simulink model "StepbyStepMotorControl_Slave_SM"  (R2018b)
settings: Solver=FixedStepDiscrete  StartTime=0.0  StopTime=10.0  FixedStep=0.1  RelTol=1e-3
InitFcn:
  | mbd_s32k14_consistency_checks(bdroot(gcs));
undefined symbols (not defined in the file): A10, AD12, AD6, AD7, Aligned, B1, B10, B8, C10, C7, C8, C9, Center, D1, D2, D8, External, G2, G3, G6, H8, K10, PTA2, PTA3, PTB10, PTB11, PTB12, PTB8, PTB9, PTC10, PTC11, PTC14, PTC6, PTC7, PTD1, PTD15, PTD16, PTD4, PTE4, PTE5, TRGMUX_PDB_TRIG
libraries: mbd_s32k14_ec_toolbox x26, simulink x2
settings Model: Creator=srjos  LastModifiedBy=srjos
settings DataIOCC: ExternalInput=off  InitialState=off  SaveOutput=off  SignalLogging=off  SaveTime=off
settings OptimizationCC: DefaultParameterBehavior=Inlined  EnhancedBackFolding=on  PassReuseOutputArgsAs=Individual arguments  OptimizeBlockOrder=speed  DifferentSizesBufferReuse=on  OptimizationCustomize=off
settings DebuggingCC: InheritedTsInSrcMsg=none  SingleTaskRateTransMsg=error  ParameterTunabilityLossMsg=error  UnconnectedInputMsg=error  UnconnectedOutputMsg=error  UnconnectedLineMsg=error  UnknownTsInhSupMsg=error
settings HardwareCC: ProdBitPerPointer=32  ProdBitPerSizeT=32  ProdBitPerPtrDiffT=32  ProdLargestAtomicInteger=Long  ProdLargestAtomicFloat=Double  ProdWordSize=32  ProdHWDeviceType=ARM Compatible->ARM Cortex
settings SFSimCC: MATLABDynamicMemAlloc=off
settings RTWCC: SystemTargetFile=mbd_s32k14.tlc  MakeCommand=mbd_s32k14_make_rtw COPY_MDLREF_INCLUDES=0  TemplateMakefile=mbd_s32k14.tmf  Description=Model Based Design Toolbox S32K14x Code Generation Target  GenerateReport=on  IncludeHyperlinkInReport=on  LaunchReport=on  GenerateTraceInfo=on  GenerateTraceReport=on  GenerateTraceReportSl=on  GenerateTraceReportSf=on  GenerateTraceReportEml=on
settings CodeAppCC: ForceParamTrailComments=on  IgnoreCustomStorageClasses=off  OperatorAnnotations=on  SimulinkDataObjDesc=on  SFDataObjDesc=on  InsertBlockDesc=on
settings STFCustomTargetCC: TargetLangStandard=C99 (ISO)  MultiwordLength=256  CombineOutputUpdateFcns=on  ERTCustomFileBanners=on  SupportContinuousTime=off  SupportNonInlinedSFcns=off  RemoveResetFunc=on  MATLABClassNameForMDSCustomization=Simulink.SoftwareTarget.ERTCustomization  SystemTargetFile=mbd_s32k14.tlc
settings ERTTargetCC: TargetLangStandard=C99 (ISO)  ParMdlRefBuildCompliant=off  CompOptLevelCompliant=off  ConcurrentExecutionCompliant=off  ModelStepFunctionPrototypeControlCompliant=off  CPPClassGenCompliant=off  UseToolchainInfoCompliant=off  InlinedParameterPlacement=NonHierarchical  ERTCustomFileTemplate=example_file_process.tlc

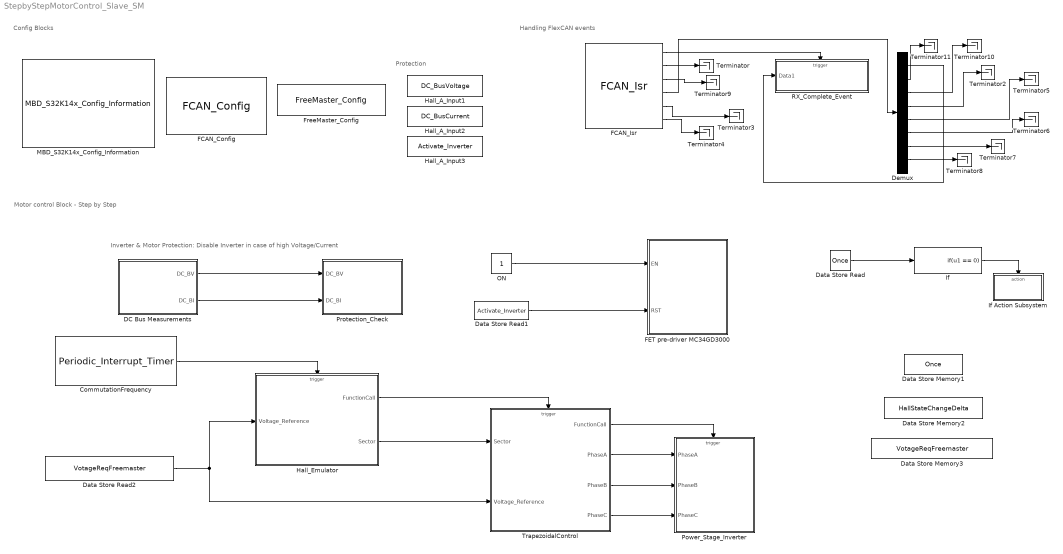
== system StepbyStepMotorControl_Slave_SM ==
  note: Config Blocks
  note: Motor control Block - Step by Step
  note: Inverter & Motor Protection: Disable Inverter in case of high Voltage/Current
  note: Protection
  note: Handling FlexCAN events
  CommutationFrequency : mbd_s32k14_ec_toolbox/S32K14x/Utility Blocks/Periodic_Interrupt_Timer  Priority=1  channel=1  chainCh=off  period=20000  prio=10  startCounter=on
  DC Bus Measurements : Subsystem  Priority=6
  Data Store Memory1 : DataStoreMemory  DataStoreName=Once  ReadBeforeWriteMsg=warning  WriteAfterWriteMsg=warning  WriteAfterReadMsg=warning  ShowAdditionalParam=off  OutDataTypeStr=uint32
  Data Store Memory2 : DataStoreMemory  DataStoreName=HallStateChangeDelta  ReadBeforeWriteMsg=warning  WriteAfterWriteMsg=warning  WriteAfterReadMsg=warning  ShowAdditionalParam=off  OutDataTypeStr=uint16
      settings: RTWStateStorageClass=ExportedGlobal
  Data Store Memory3 : DataStoreMemory  DataStoreName=VotageReqFreemaster  ReadBeforeWriteMsg=warning  WriteAfterWriteMsg=warning  WriteAfterReadMsg=warning  ShowAdditionalParam=off  OutDataTypeStr=int16
      settings: RTWStateStorageClass=ExportedGlobal
  Data Store Read : DataStoreRead  DataStoreName=Once
  Data Store Read1 : DataStoreRead  DataStoreName=Activate_Inverter
  Data Store Read2 : DataStoreRead  DataStoreName=VotageReqFreemaster
  Demux : Demux  Outputs=8
  FCAN_Config : mbd_s32k14_ec_toolbox/S32K14x/Communication Blocks/Flex CAN Blocks/FCAN_Config  Priority=1  can_instance=0  can_mode=Normal mode  can_max_num_mb=16  can_rx=PTE4 : [9] : [6] : [D1]  can_tx=PTE5 : [8] : [5] : [D2]  show_adv_opts=on  can_clk_src=Peripheral clock  can_presdiv=9  can_rjw=0  can_pseg1=3  can_pseg2=3  can_propseg=6  can_cbt_presdiv=9  can_cbt_rjw=0  can_cbt_pseg1=3  can_cbt_pseg2=3  can_cbt_propseg=6  can_fd_enable=on  can_payload=8  can_rxfifo_enable=off  can_fifo_id_filter_extended=off  can_fifo_id_filter_remote=off  can_num_id_filters=8  can_fifo_id_format=A  can_fifo_id_filter={'0x0', '0x0', '0x0', '0x0', '0x0', '0x0', '0x0', '0x0'}  can_pn_enable=off  can_wakeup_match=off  can_wakeup_timeout=off  can_timeout_en=off  can_match_timeout=1  can_multiple_matches_en=off  can_num_matches=1  can_idfilter_extendedid=off  can_idfilter_remoteframe=off  can_idfilter_type=Match exact  can_idfilter_id1=0  can_idfilter_id2=0  can_payloadfilter_enable=off  can_payloadfilter_dlclow=0  can_payloadfilter_dlchigh=0  can_payloadfilter_type=Match exact  can_payloadfilter_payload1_b0=0  can_payloadfilter_payload1_b1=0  can_payloadfilter_payload1_b2=0  can_payloadfilter_payload1_b3=0  can_payloadfilter_payload1_b4=0  can_payloadfilter_payload1_b5=0  can_payloadfilter_payload1_b6=0  can_payloadfilter_payload1_b7=0  can_payloadfilter_payload2_b0=0  can_payloadfilter_payload2_b1=0  can_payloadfilter_payload2_b2=0  can_payloadfilter_payload2_b3=0  can_payloadfilter_payload2_b4=0  can_payloadfilter_payload2_b5=0  can_payloadfilter_payload2_b6=0  can_payloadfilter_payload2_b7=0
  FCAN_Isr : mbd_s32k14_ec_toolbox/S32K14x/Communication Blocks/Flex CAN Blocks/FCAN_Isr  can_instance=0  can_event=Rx Complete
  FET pre-driver MC34GD3000 : Subsystem
  FreeMaster_Config : mbd_s32k14_ec_toolbox/S32K14x/Utility Blocks/FreeMaster_Config  interface=UART1  baudrate=115200  rxd=PTC6 : [81] : [52] : [C7]  txd=PTC7 : [80] : [51] : [B8]  mode=Short Interrupt  isr_prio=15  show_adv_opts=off  use_scope=on  max_scope_vars=8  use_recorder=on  max_rec_vars=8  rec_buff_size=1024  rec_timebase=0 milliseconds  comm_buffer_size_auto=on  comm_buffer_size=255  comm_rqueue_size_default=on  comm_rqueue_size=32
  Hall_A_Input1 : DataStoreMemory  DataStoreName=DC_BusVoltage  ReadBeforeWriteMsg=warning  WriteAfterWriteMsg=warning  WriteAfterReadMsg=warning  ShowAdditionalParam=off  OutDataTypeStr=single
  Hall_A_Input2 : DataStoreMemory  DataStoreName=DC_BusCurrent  ReadBeforeWriteMsg=warning  WriteAfterWriteMsg=warning  WriteAfterReadMsg=warning  ShowAdditionalParam=off  OutDataTypeStr=single
  Hall_A_Input3 : DataStoreMemory  DataStoreName=Activate_Inverter  ReadBeforeWriteMsg=warning  WriteAfterWriteMsg=warning  WriteAfterReadMsg=warning  ShowAdditionalParam=off  OutDataTypeStr=boolean
  Hall_Emulator : Subsystem
      settings: PropExecContextOutsideSubsystem=on  RTWSystemCode=Nonreusable function
  If : If  IfExpression=u1 == 0  ShowElse=off
  If Action Subsystem : Subsystem  TreatAsAtomicUnit=on
  MBD_S32K14x_Config_Information : mbd_s32k14_ec_toolbox/S32K14x/MBD_S32K14x_Config_Information  disp_str=|  config_params=[]
      | Target : S32K144-64KB_SRAM
      | Package : 100-pin
      | System clock : 80 MHz
      | XTAL clock : External 8 MHz
      | Compiler : GCC
      | Target Type : FLASH
      | Download Code after build : (OpenSDA: E)
      | Step Tick Interrupt Priority : 15
  ON : Constant  OutDataTypeStr=boolean
  Power_Stage_Inverter : Subsystem  TreatAsAtomicUnit=on
      settings: RTWSystemCode=Nonreusable function
  Protection_Check : Subsystem
  RX_Complete_Event : Subsystem  TreatAsAtomicUnit=on
      settings: RTWSystemCode=Nonreusable function
  Terminator{,2..11} (11 alike) : Terminator
  TrapezoidalControl : Subsystem
      settings: RTWSystemCode=Nonreusable function
  wires:
  DC Bus Measurements/2(DC_BI) -> Protection_Check/2(DC_BI)
  CommutationFrequency/1 -> Hall_Emulator/Trigger
  Data Store Read1/1 -> FET pre-driver MC34GD3000/2(RST)
  DC Bus Measurements/1(DC_BV) -> Protection_Check/1(DC_BV)
  TrapezoidalControl/1(FunctionCall) -> Power_Stage_Inverter/Trigger
  TrapezoidalControl/2(PhaseA) -> Power_Stage_Inverter/1(PhaseA)
  Data Store Read2/1 -> TrapezoidalControl/2(Voltage_Reference), Hall_Emulator/1(Voltage_Reference)
  ON/1 -> FET pre-driver MC34GD3000/1(EN)
  TrapezoidalControl/4(PhaseC) -> Power_Stage_Inverter/3(PhaseC)
  Hall_Emulator/1(FunctionCall) -> TrapezoidalControl/Trigger
  TrapezoidalControl/3(PhaseB) -> Power_Stage_Inverter/2(PhaseB)
  Hall_Emulator/2(Sector) -> TrapezoidalControl/1(Sector)
  Demux/4 -> Terminator2/1
  FCAN_Isr/4 -> Demux/1
  FCAN_Isr/2 -> Terminator/1
  FCAN_Isr/6 -> Terminator4/1
  FCAN_Isr/1 -> RX_Complete_Event/Trigger
  Demux/5 -> Terminator5/1
  Demux/7 -> Terminator7/1
  Demux/1 -> RX_Complete_Event/1(Data1)
  FCAN_Isr/3 -> Terminator9/1
  Demux/6 -> Terminator6/1
  Demux/2 -> Terminator11/1
  Demux/3 -> Terminator10/1
  Demux/8 -> Terminator8/1
  FCAN_Isr/5 -> Terminator3/1
  If/1 -> If Action Subsystem/Action
  Data Store Read/1 -> If/1

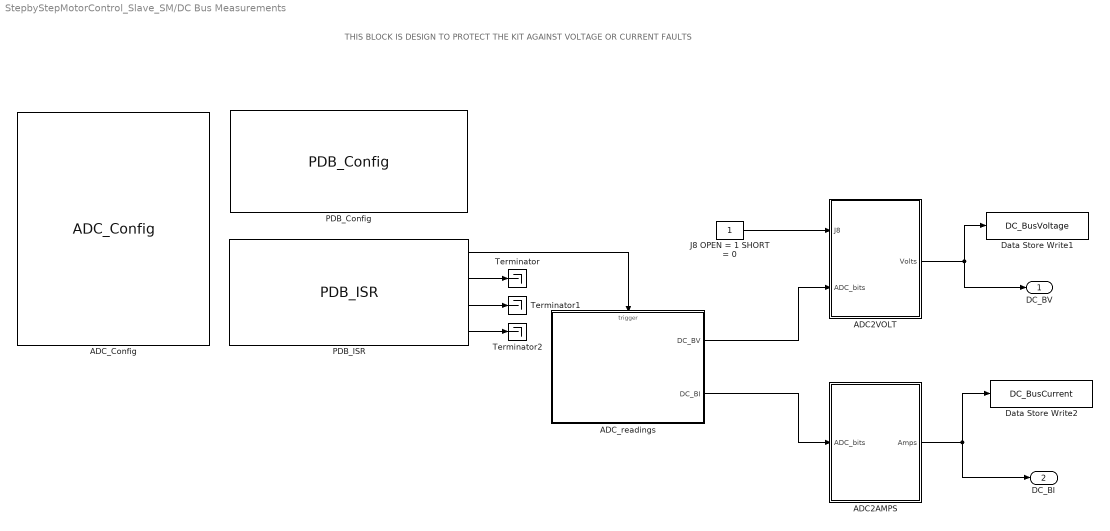
== system StepbyStepMotorControl_Slave_SM/DC Bus Measurements ==
  note: THIS BLOCK IS DESIGN TO PROTECT THE KIT AGAINST VOLTAGE OR CURRENT FAULTS
  ADC2AMPS : Subsystem
  ADC2VOLT : Subsystem
  ADC_Config : mbd_s32k14_ec_toolbox/S32K14x/Motor Control Blocks/ADC Blocks/ADC_Config  Priority=1  instance=1  mode=12-bit conversion  smplts=64  adiclk=alternate clock 1  adiv=input clock  show_adv_opts=on  pretrgsel=PDB pre-trigger  swpretrg=Disabled  adtrg=hardware  trgsel=PDB output  refsel=Vrefh and Vrefl  acfe=off  acfgt=off  acren=off  cv1=0  cv2=0  adco=off  avge=off  avgs=16 samples
  ADC_readings : Subsystem  TreatAsAtomicUnit=on
      settings: RTWSystemCode=Nonreusable function
  Data Store Write1 : DataStoreWrite  DataStoreName=DC_BusVoltage
  Data Store Write2 : DataStoreWrite  DataStoreName=DC_BusCurrent
  J8 OPEN = 1 SHORT = 0 : Constant  OutDataTypeStr=boolean
  PDB_Config : mbd_s32k14_ec_toolbox/S32K14x/Motor Control Blocks/PDB Blocks/PDB_Config  Priority=1  pdbModule=1  regScCont=Continuous  regScTrgsel=External (TRGMUX_PDB_TRIG)  trgMuxSel=FTM3 External Trigger  regModModulus=10000  regScPrescaler=8  regScMult=1  regPoenPoen0=off  regPo0DlyDly1=0  regPo0DlyDly2=1000  show_adv_opts=off  regCh0C1En0=on  regCh0C1En1=on  regCh0C1En2=off  regCh0C1En3=off  regCh0C1En4=off  regCh0C1En5=off  regCh0C1En6=off  regCh0C1En7=off  regCh0C1Bb0=off  regCh0C1Bb1=off  regCh0C1Bb2=off  regCh0C1Bb3=off  regCh0C1Bb4=off  regCh0C1Bb5=off  regCh0C1Bb6=off  regCh0C1Bb7=off  regCh0C1Tos0=Pre-trigger is in delay mode  regCh0C1Tos1=Pre-trigger is in delay mode  regCh0C1Tos2=Pre-trigger is in delay mode  regCh0C1Tos3=Pre-trigger is in delay mode  regCh0C1Tos4=Pre-trigger is in delay mode  regCh0C1Tos5=Pre-trigger is in delay mode  regCh0C1Tos6=Pre-trigger is in delay mode  regCh0C1Tos7=Pre-trigger is in delay mode  regCh0DlyDly0=300  regCh0DlyDly1=400  regCh0DlyDly2=100  regCh0DlyDly3=480  regCh0DlyDly4=600  regCh0DlyDly5=720  regCh0DlyDly6=840  regCh0DlyDly7=960  regCh1C1En0=off  regCh1C1En1=off  regCh1C1En2=off  regCh1C1En3=off  regCh1C1En4=off  regCh1C1En5=off  regCh1C1En6=off  regCh1C1En7=off  regCh1C1Bb0=off  regCh1C1Bb1=off  regCh1C1Bb2=off  regCh1C1Bb3=off  regCh1C1Bb4=off  regCh1C1Bb5=off  regCh1C1Bb6=off  regCh1C1Bb7=off  regCh1C1Tos0=Pre-trigger is in delay mode  regCh1C1Tos1=Pre-trigger is in delay mode  regCh1C1Tos2=Pre-trigger is in delay mode  regCh1C1Tos3=Pre-trigger is in delay mode  regCh1C1Tos4=Pre-trigger is in delay mode  regCh1C1Tos5=Pre-trigger is in delay mode  regCh1C1Tos6=Pre-trigger is in delay mode  regCh1C1Tos7=Pre-trigger is in delay mode  regCh1DlyDly0=100  regCh1DlyDly1=200  regCh1DlyDly2=300  regCh1DlyDly3=400  regCh1DlyDly4=500  regCh1DlyDly5=600  regCh1DlyDly6=700  regCh1DlyDly7=800
  PDB_ISR : mbd_s32k14_ec_toolbox/S32K14x/Motor Control Blocks/PDB Blocks/PDB_ISR  Priority=2  pdbModule=1  prioInterrupt=5  regScPdbie=on  regScPdbeie=off  regIdlyIdly=0
  Terminator : Terminator
  Terminator1 : Terminator
  Terminator2 : Terminator
  DC_BV : Outport
  DC_BI : Outport  Port=2
  wires:
  PDB_ISR/2 -> Terminator/1
  PDB_ISR/4 -> Terminator2/1
  PDB_ISR/3 -> Terminator1/1
  PDB_ISR/1 -> ADC_readings/Trigger
  ADC2VOLT/1(Volts) -> DC_BV/1, Data Store Write1/1
  J8 OPEN = 1 SHORT = 0/1 -> ADC2VOLT/1(J8)
  ADC_readings/1(DC_BV) -> ADC2VOLT/2(ADC_bits)
  ADC2AMPS/1(Amps) -> Data Store Write2/1, DC_BI/1
  ADC_readings/2(DC_BI) -> ADC2AMPS/1(ADC_bits)

== system StepbyStepMotorControl_Slave_SM/FET pre-driver MC34GD3000 ==
  EN : Inport
  RST : Inport  Port=2
  GD3000_EN : mbd_s32k14_ec_toolbox/S32K14x/Peripheral Interface Blocks/Digital_Output  gpio_pin=PTA2 : [73] : [48] : [C10]  port=A  pin=2  drive_strength=High  slew_rate=Fast
  GD3000_RST : mbd_s32k14_ec_toolbox/S32K14x/Peripheral Interface Blocks/Digital_Output  gpio_pin="PTA3 : [72] : [47]  : [D8]"  port=A  pin=3  drive_strength=High  slew_rate=Fast
  wires:
  EN/1 -> GD3000_EN/1
  RST/1 -> GD3000_RST/1

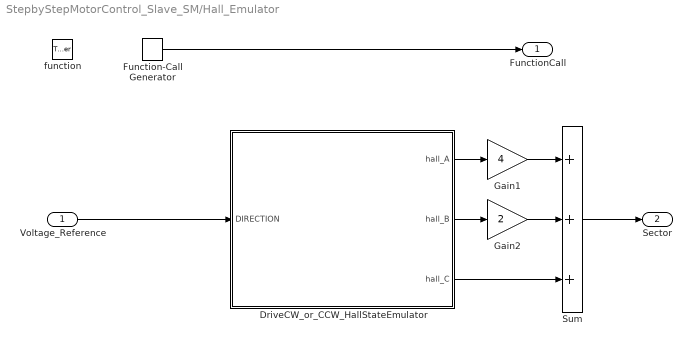
== system StepbyStepMotorControl_Slave_SM/Hall_Emulator ==
  Voltage_Reference : Inport
  function : TriggerPort  TriggerType=function-call  VariantControl=(inherit)
  DriveCW_or_CCW_HallStateEmulator : Stateflow chart  TreatAsAtomicUnit=on
  Function-Call Generator : simulink/Ports & Subsystems/Function-Call Generator  sample_time=-1  numberOfIterations=1
  Gain1 : Gain  Gain=4  OutDataTypeStr=uint8  ParamDataTypeStr=Inherit: Same as input
  Gain2 : Gain  Gain=2  OutDataTypeStr=uint8  ParamDataTypeStr=Inherit: Same as input
  Sum : Sum  Inputs=+++  AccumDataTypeStr=uint8  OutDataTypeStr=uint8
  FunctionCall : Outport
  Sector : Outport  Port=2  OutDataTypeStr=uint8
  wires:
  Function-Call Generator/1 -> FunctionCall/1
  Gain1/1 -> Sum/1
  DriveCW_or_CCW_HallStateEmulator/1(hall_A) -> Gain1/1
  Gain2/1 -> Sum/2
  DriveCW_or_CCW_HallStateEmulator/3(hall_C) -> Sum/3
  DriveCW_or_CCW_HallStateEmulator/2(hall_B) -> Gain2/1
  Sum/1 -> Sector/1
  Voltage_Reference/1 -> DriveCW_or_CCW_HallStateEmulator/1(DIRECTION)

== system StepbyStepMotorControl_Slave_SM/If Action Subsystem ==
  Action Port : ActionPort  ActionType=then
  Constant : Constant  OutDataTypeStr=uint32
  Data Store Write : DataStoreWrite  DataStoreName=Once
  FCAN_Receive_ID_0x3FF : mbd_s32k14_ec_toolbox/S32K14x/Communication Blocks/Flex CAN Blocks/FCAN_Receive  can_instance=0  can_mode=Non-blocking  can_timeout_ms=0  can_mb_idx=14  can_extended_id=off  can_is_remote=off  can_id=3FF  can_msg_mask=FFFFFFFF  show_adv_opts=on  can_use_rxfifo=off  can_fd_enable=on
  wires:
  Constant/1 -> Data Store Write/1

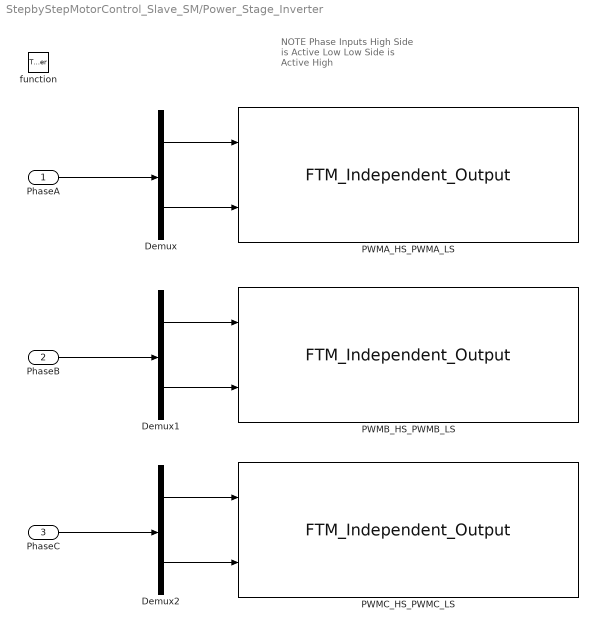
== system StepbyStepMotorControl_Slave_SM/Power_Stage_Inverter ==
  note: NOTE
      | Phase Inputs
      | High Side is Active Low
      | Low Side is Active High
  PhaseA : Inport
  PhaseB : Inport  Port=2
  PhaseC : Inport  Port=3
  function : TriggerPort  TriggerType=function-call  VariantControl=(inherit)
  Demux : Demux  Outputs=2
  Demux1 : Demux  Outputs=2
  Demux2 : Demux  Outputs=2
  PWMA_HS_PWMA_LS : mbd_s32k14_ec_toolbox/S32K14x/Motor Control Blocks/FlexTimer Blocks/FTM_Independent_Output  ftmModule=3  channelPair=0-1  pwmMode=Center-Aligned  outFrequency=5000  resolution=1 %  dutyCycleChN=50  dutyCycleChNP1=0  dutyCycleSim=off  startAfterInit=on  showAdvOpt=off  pinFtm0Ch0=None  pinFtm0Ch1=None  pinFtm0Ch2=None  pinFtm0Ch3=None  pinFtm0Ch4=None  pinFtm0Ch5=None  pinFtm0Ch6=None  pinFtm0Ch7=None  pinFtm1Ch0=None  pinFtm1Ch1=None  pinFtm1Ch2=None  pinFtm1Ch3=None  pinFtm1Ch4=None  pinFtm1Ch5=None  pinFtm1Ch6=None  pinFtm1Ch7=None  pinFtm2Ch0=None  pinFtm2Ch1=None  pinFtm2Ch2=None  pinFtm2Ch3=None  pinFtm2Ch4=None  pinFtm2Ch5=None  pinFtm2Ch6=None  pinFtm2Ch7=None  pinFtm3Ch0=PTB8 : [77] : [---] : [A10]  pinFtm3Ch1=PTB9 : [76] : [---] : [C8]  pinFtm3Ch2=None  pinFtm3Ch3=None  pinFtm3Ch4=None  pinFtm3Ch5=None  pinFtm3Ch6=None  pinFtm3Ch7=None  outputLevelN=Low-true pulses  outputLevelNP1=High-true pulses  initTrigger=on  chNTrigger=off  chNP1Trigger=on  mcuTargetUpdate=on
  PWMB_HS_PWMB_LS : mbd_s32k14_ec_toolbox/S32K14x/Motor Control Blocks/FlexTimer Blocks/FTM_Independent_Output  ftmModule=3  channelPair=2-3  pwmMode=Center-Aligned  outFrequency=5000  resolution=1 %  dutyCycleChN=50  dutyCycleChNP1=0  dutyCycleSim=off  startAfterInit=on  showAdvOpt=off  pinFtm0Ch0=None  pinFtm0Ch1=None  pinFtm0Ch2=None  pinFtm0Ch3=None  pinFtm0Ch4=None  pinFtm0Ch5=None  pinFtm0Ch6=None  pinFtm0Ch7=None  pinFtm1Ch0=None  pinFtm1Ch1=None  pinFtm1Ch2=None  pinFtm1Ch3=None  pinFtm1Ch4=None  pinFtm1Ch5=None  pinFtm1Ch6=None  pinFtm1Ch7=None  pinFtm2Ch0=None  pinFtm2Ch1=None  pinFtm2Ch2=None  pinFtm2Ch3=None  pinFtm2Ch4=None  pinFtm2Ch5=None  pinFtm2Ch6=None  pinFtm2Ch7=None  pinFtm3Ch0=PTB8 : [77] : [---] : [A10]  pinFtm3Ch1=PTB9 : [76] : [---] : [C8]  pinFtm3Ch2=PTB10 : [75] : [---] : [B10]  pinFtm3Ch3=PTB11 : [74] : [---] : [C9]  pinFtm3Ch4=None  pinFtm3Ch5=None  pinFtm3Ch6=None  pinFtm3Ch7=None  outputLevelN=Low-true pulses  outputLevelNP1=High-true pulses  initTrigger=off  chNTrigger=off  chNP1Trigger=off  mcuTargetUpdate=on
  PWMC_HS_PWMC_LS : mbd_s32k14_ec_toolbox/S32K14x/Motor Control Blocks/FlexTimer Blocks/FTM_Independent_Output  ftmModule=3  channelPair=4-5  pwmMode=Center-Aligned  outFrequency=5000  resolution=1 %  dutyCycleChN=50  dutyCycleChNP1=0  dutyCycleSim=off  startAfterInit=on  showAdvOpt=off  pinFtm0Ch0=None  pinFtm0Ch1=None  pinFtm0Ch2=None  pinFtm0Ch3=None  pinFtm0Ch4=None  pinFtm0Ch5=None  pinFtm0Ch6=None  pinFtm0Ch7=None  pinFtm1Ch0=None  pinFtm1Ch1=None  pinFtm1Ch2=None  pinFtm1Ch3=None  pinFtm1Ch4=None  pinFtm1Ch5=None  pinFtm1Ch6=None  pinFtm1Ch7=None  pinFtm2Ch0=None  pinFtm2Ch1=None  pinFtm2Ch2=None  pinFtm2Ch3=None  pinFtm2Ch4=None  pinFtm2Ch5=None  pinFtm2Ch6=None  pinFtm2Ch7=None  pinFtm3Ch0=PTB8 : [77] : [---] : [A10]  pinFtm3Ch1=PTB9 : [76] : [---] : [C8]  pinFtm3Ch2=PTB10 : [75] : [---] : [B10]  pinFtm3Ch3=PTB11 : [74] : [---] : [C9]  pinFtm3Ch4=PTC10 : [52] : [---] : [K10]  pinFtm3Ch5=PTC11 : [51] : [---] : [H8]  pinFtm3Ch6=None  pinFtm3Ch7=None  outputLevelN=Low-true pulses  outputLevelNP1=High-true pulses  initTrigger=off  chNTrigger=off  chNP1Trigger=off  mcuTargetUpdate=on
  wires:
  Demux/1 -> PWMA_HS_PWMA_LS/1
  Demux/2 -> PWMA_HS_PWMA_LS/2
  PhaseA/1 -> Demux/1
  PhaseB/1 -> Demux1/1
  Demux1/1 -> PWMB_HS_PWMB_LS/1
  Demux1/2 -> PWMB_HS_PWMB_LS/2
  PhaseC/1 -> Demux2/1
  Demux2/1 -> PWMC_HS_PWMC_LS/1
  Demux2/2 -> PWMC_HS_PWMC_LS/2

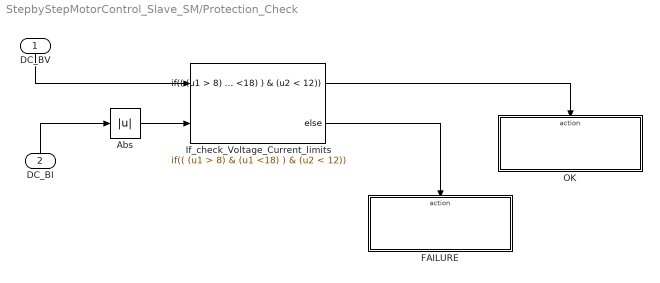
== system StepbyStepMotorControl_Slave_SM/Protection_Check ==
  DC_BV : Inport
  DC_BI : Inport  Port=2
  Abs : Abs
  FAILURE : Subsystem  TreatAsAtomicUnit=on
  If_check_Voltage_Current_limits : If  NumInputs=2  IfExpression=( (u1 > 8) & (u1 <18) ) & (u2 < 12)
  OK : Subsystem  TreatAsAtomicUnit=on
  wires:
  DC_BV/1 -> If_check_Voltage_Current_limits/1
  Abs/1 -> If_check_Voltage_Current_limits/2
  DC_BI/1 -> Abs/1
  If_check_Voltage_Current_limits/1 -> OK/Action
  If_check_Voltage_Current_limits/2 -> FAILURE/Action

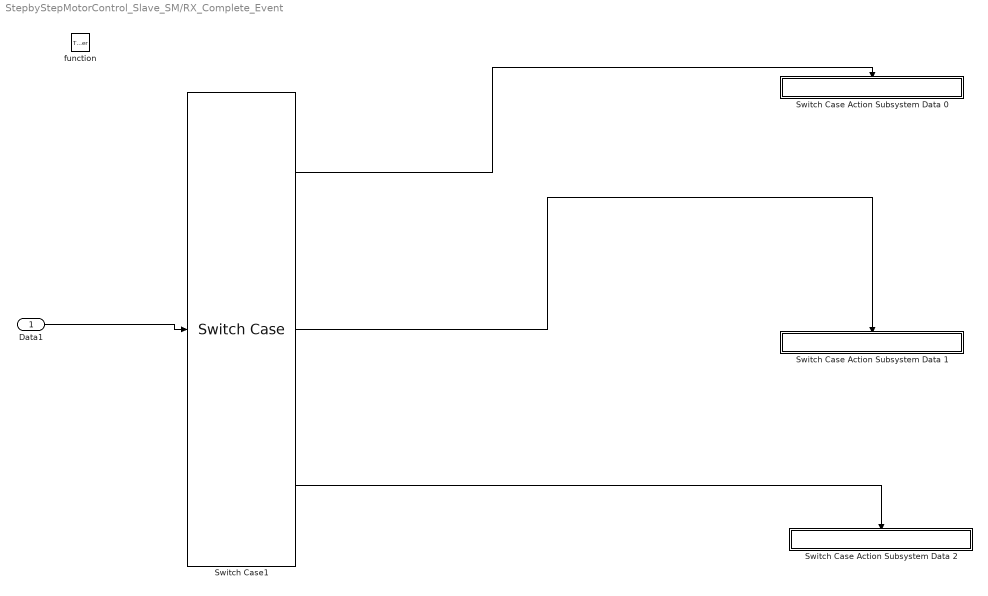
== system StepbyStepMotorControl_Slave_SM/RX_Complete_Event ==
  Data1 : Inport
  function : TriggerPort  TriggerType=function-call  VariantControl=(inherit)
  Switch Case Action Subsystem Data 0 : Subsystem  TreatAsAtomicUnit=on
  Switch Case Action Subsystem Data 1 : Subsystem  TreatAsAtomicUnit=on
  Switch Case Action Subsystem Data 2 : Subsystem  TreatAsAtomicUnit=on
  Switch Case1 : SwitchCase  CaseConditions={hex2dec('030'),hex2dec('031'), hex2dec('032')}  ShowDefaultCase=off
  wires:
  Switch Case1/1 -> Switch Case Action Subsystem Data 0/Action
  Switch Case1/2 -> Switch Case Action Subsystem Data 1/Action
  Data1/1 -> Switch Case1/1
  Switch Case1/3 -> Switch Case Action Subsystem Data 2/Action

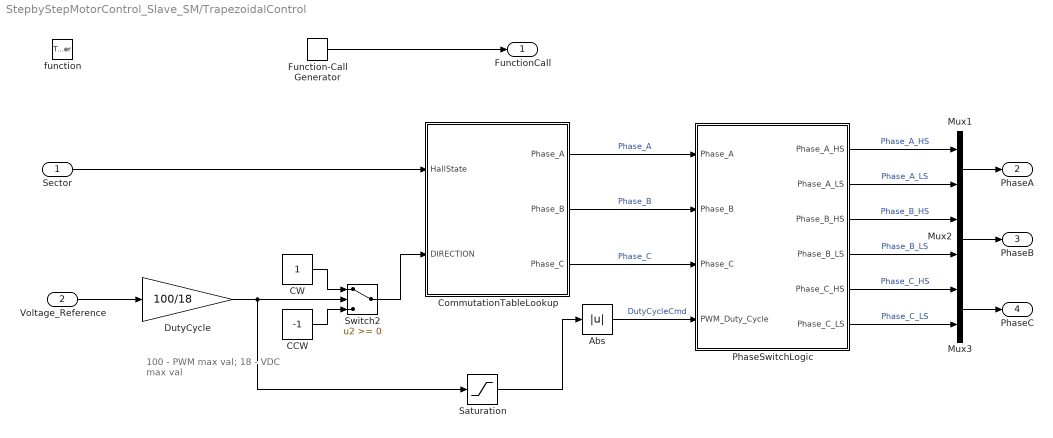
== system StepbyStepMotorControl_Slave_SM/TrapezoidalControl ==
  note: 100 - PWM max val;
      | 18  -  VDC max val
  Sector : Inport
  Voltage_Reference : Inport  Port=2
  function : TriggerPort  TriggerType=function-call  VariantControl=(inherit)
  Abs : Abs  OutMin=0  OutMax=100  OutDataTypeStr=Inherit: Inherit via internal rule
  CCW : Constant  Value=-1  OutDataTypeStr=single
  CW : Constant  OutDataTypeStr=single
  CommutationTableLookup : Stateflow chart  TreatAsAtomicUnit=on
  DutyCycle : Gain  Gain=100/18  OutMin=-100  OutMax=100  OutDataTypeStr=single  ParamDataTypeStr=Inherit: Same as input
  Function-Call Generator : simulink/Ports & Subsystems/Function-Call Generator  sample_time=-1  numberOfIterations=1
  Mux1 : Mux  Inputs=2
  Mux2 : Mux  Inputs=2
  Mux3 : Mux  Inputs=2
  PhaseSwitchLogic : Stateflow chart  TreatAsAtomicUnit=on
  Saturation : Saturate  UpperLimit=100  LowerLimit=-100
  Switch2 : Switch  OutDataTypeStr=single
  FunctionCall : Outport
  PhaseA : Outport  Port=2
  PhaseB : Outport  Port=3
  PhaseC : Outport  Port=4
  wires:
  Function-Call Generator/1 -> FunctionCall/1
  Mux1/1 -> PhaseA/1
  CommutationTableLookup/1(Phase_A) -> PhaseSwitchLogic/1(Phase_A)  "Phase_A"
  CommutationTableLookup/2(Phase_B) -> PhaseSwitchLogic/2(Phase_B)  "Phase_B"
  CommutationTableLookup/3(Phase_C) -> PhaseSwitchLogic/3(Phase_C)  "Phase_C"
  PhaseSwitchLogic/1(Phase_A_HS) -> Mux1/1  "Phase_A_HS"
  PhaseSwitchLogic/2(Phase_A_LS) -> Mux1/2  "Phase_A_LS"
  PhaseSwitchLogic/3(Phase_B_HS) -> Mux2/1  "Phase_B_HS"
  PhaseSwitchLogic/4(Phase_B_LS) -> Mux2/2  "Phase_B_LS"
  PhaseSwitchLogic/5(Phase_C_HS) -> Mux3/1  "Phase_C_HS"
  PhaseSwitchLogic/6(Phase_C_LS) -> Mux3/2  "Phase_C_LS"
  CW/1 -> Switch2/1
  CCW/1 -> Switch2/3
  Voltage_Reference/1 -> DutyCycle/1
  Abs/1 -> PhaseSwitchLogic/4(PWM_Duty_Cycle)  "DutyCycleCmd"
  Switch2/1 -> CommutationTableLookup/2(DIRECTION)
  DutyCycle/1 -> Switch2/2, Saturation/1
  Sector/1 -> CommutationTableLookup/1(HallState)
  Mux2/1 -> PhaseB/1
  Mux3/1 -> PhaseC/1
  Saturation/1 -> Abs/1

== system StepbyStepMotorControl_Slave_SM/DC Bus Measurements/ADC2AMPS ==
  ADC_bits : Inport
  Sum : Sum  Inputs=+-  OutDataTypeStr=single
  bits2amps : Gain  Gain=25/4095  OutDataTypeStr=single
  offset : Constant  Value=2048  OutDataTypeStr=uint32
  Amps : Outport
  wires:
  Sum/1 -> bits2amps/1
  bits2amps/1 -> Amps/1
  offset/1 -> Sum/2
  ADC_bits/1 -> Sum/1

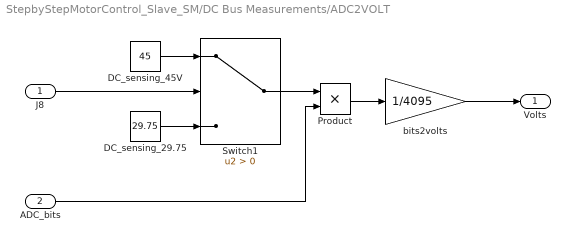
== system StepbyStepMotorControl_Slave_SM/DC Bus Measurements/ADC2VOLT ==
  J8 : Inport
  ADC_bits : Inport  Port=2
  DC_sensing_29.75 : Constant  Value=29.75  OutDataTypeStr=single
  DC_sensing_45V : Constant  Value=45  OutDataTypeStr=single
  Product : Product  OutDataTypeStr=single
  Switch1 : Switch  Criteria=u2 > Threshold
  bits2volts : Gain  Gain=1/4095  OutDataTypeStr=single
  Volts : Outport
  wires:
  bits2volts/1 -> Volts/1
  DC_sensing_45V/1 -> Switch1/1
  DC_sensing_29.75/1 -> Switch1/3
  Product/1 -> bits2volts/1
  J8/1 -> Switch1/2
  Switch1/1 -> Product/1
  ADC_bits/1 -> Product/2

== system StepbyStepMotorControl_Slave_SM/DC Bus Measurements/ADC_readings ==
  function : TriggerPort  TriggerType=function-call  VariantControl=(inherit)
  Read_DC_Current : mbd_s32k14_ec_toolbox/S32K14x/Motor Control Blocks/ADC Blocks/ADC_Start  instance=1  adc_r=B  adc0_chan=PTC14 : [46] : [30] : [G6] : AD12  adc1_chan=PTD4 : [69] : [44] : [E10] : AD6  aien=off  mcuTargetUpdate=on
  Read_DC_Voltage : mbd_s32k14_ec_toolbox/S32K14x/Motor Control Blocks/ADC Blocks/ADC_Start  instance=1  adc_r=A  adc0_chan=PTC14 : [46] : [30] : [G6] : AD12  adc1_chan=PTB12 : [68] : [43] : [E9] : AD7  aien=off  mcuTargetUpdate=on
  DC_BV : Outport
  DC_BI : Outport  Port=2
  wires:
  Read_DC_Voltage/1 -> DC_BV/1
  Read_DC_Current/1 -> DC_BI/1

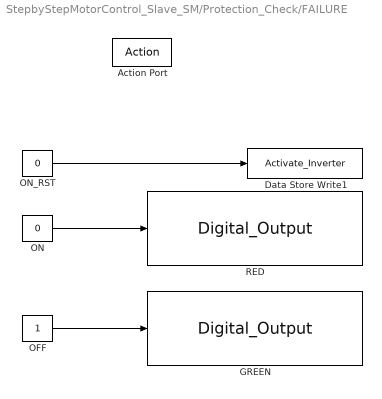
== system StepbyStepMotorControl_Slave_SM/Protection_Check/FAILURE ==
  Action Port : ActionPort  ActionType=else
  Data Store Write1 : DataStoreWrite  DataStoreName=Activate_Inverter
  GREEN : mbd_s32k14_ec_toolbox/S32K14x/Peripheral Interface Blocks/Digital_Output  gpio_pin=PTD16 : [21] : [14] : [G2]  port=D  pin=16  drive_strength=Low  slew_rate=Fast
  OFF : Constant  OutDataTypeStr=boolean
  ON : Constant  Value=0  OutDataTypeStr=boolean
  ON_RST : Constant  Value=0  OutDataTypeStr=boolean
  RED : mbd_s32k14_ec_toolbox/S32K14x/Peripheral Interface Blocks/Digital_Output  gpio_pin=PTD15 : [22] : [15] : [G3]  port=D  pin=15  drive_strength=Low  slew_rate=Fast
  wires:
  ON/1 -> RED/1
  ON_RST/1 -> Data Store Write1/1
  OFF/1 -> GREEN/1

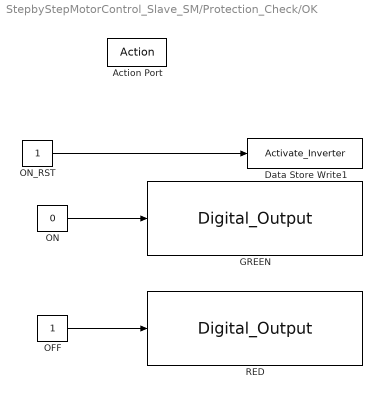
== system StepbyStepMotorControl_Slave_SM/Protection_Check/OK ==
  Action Port : ActionPort  ActionType=then
  Data Store Write1 : DataStoreWrite  DataStoreName=Activate_Inverter
  GREEN : mbd_s32k14_ec_toolbox/S32K14x/Peripheral Interface Blocks/Digital_Output  gpio_pin=PTD16 : [21] : [14] : [G2]  port=D  pin=16  drive_strength=Low  slew_rate=Fast
  OFF : Constant  OutDataTypeStr=boolean
  ON : Constant  Value=0  OutDataTypeStr=boolean
  ON_RST : Constant  OutDataTypeStr=boolean
  RED : mbd_s32k14_ec_toolbox/S32K14x/Peripheral Interface Blocks/Digital_Output  gpio_pin=PTD15 : [22] : [15] : [G3]  port=D  pin=15  drive_strength=Low  slew_rate=Fast
  wires:
  ON/1 -> GREEN/1
  ON_RST/1 -> Data Store Write1/1
  OFF/1 -> RED/1

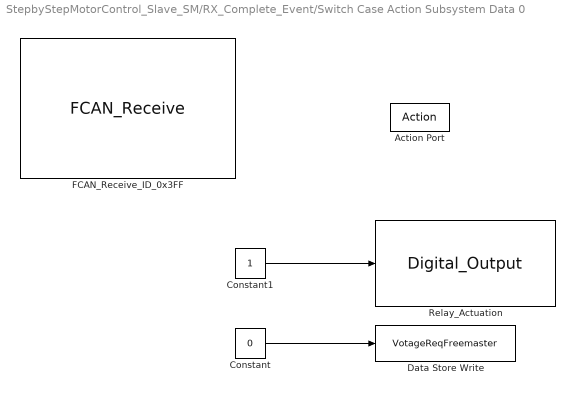
== system StepbyStepMotorControl_Slave_SM/RX_Complete_Event/Switch Case Action Subsystem Data 0 ==
  Action Port : ActionPort  ActionType=case
  Constant : Constant  Value=0  OutDataTypeStr=int16
  Constant1 : Constant  OutDataTypeStr=boolean
  Data Store Write : DataStoreWrite  DataStoreName=VotageReqFreemaster
  FCAN_Receive_ID_0x3FF : mbd_s32k14_ec_toolbox/S32K14x/Communication Blocks/Flex CAN Blocks/FCAN_Receive  can_instance=0  can_mode=Non-blocking  can_timeout_ms=0  can_mb_idx=14  can_extended_id=off  can_is_remote=off  can_id=3FF  can_msg_mask=FFFFFFFF  show_adv_opts=on  can_use_rxfifo=off  can_fd_enable=on
  Relay_Actuation : mbd_s32k14_ec_toolbox/S32K14x/Peripheral Interface Blocks/Digital_Output  gpio_pin=PTD1 : [3] : [1] : [B1]  port=D  pin=1  drive_strength=Low  slew_rate=Fast
  wires:
  Constant/1 -> Data Store Write/1
  Constant1/1 -> Relay_Actuation/1

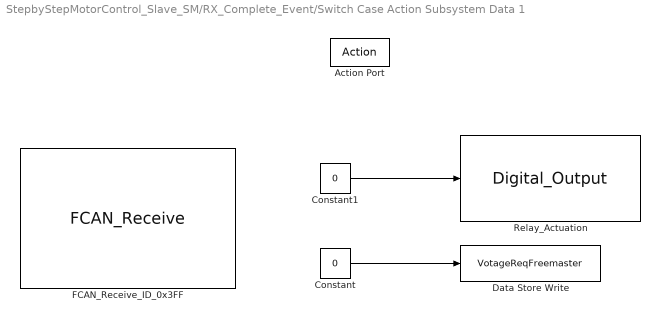
== system StepbyStepMotorControl_Slave_SM/RX_Complete_Event/Switch Case Action Subsystem Data 1 ==
  Action Port : ActionPort  ActionType=case
  Constant : Constant  Value=0  OutDataTypeStr=int16
  Constant1 : Constant  Value=0  OutDataTypeStr=boolean
  Data Store Write : DataStoreWrite  DataStoreName=VotageReqFreemaster
  FCAN_Receive_ID_0x3FF : mbd_s32k14_ec_toolbox/S32K14x/Communication Blocks/Flex CAN Blocks/FCAN_Receive  can_instance=0  can_mode=Non-blocking  can_timeout_ms=0  can_mb_idx=14  can_extended_id=off  can_is_remote=off  can_id=3FF  can_msg_mask=FFFFFFFF  show_adv_opts=on  can_use_rxfifo=off  can_fd_enable=on
  Relay_Actuation : mbd_s32k14_ec_toolbox/S32K14x/Peripheral Interface Blocks/Digital_Output  gpio_pin=PTD1 : [3] : [1] : [B1]  port=D  pin=1  drive_strength=Low  slew_rate=Fast
  wires:
  Constant/1 -> Data Store Write/1
  Constant1/1 -> Relay_Actuation/1

== system StepbyStepMotorControl_Slave_SM/RX_Complete_Event/Switch Case Action Subsystem Data 2 ==
  Action Port : ActionPort  ActionType=case
  Constant : Constant  Value=8  OutDataTypeStr=int16
  Constant1 : Constant  Value=0  OutDataTypeStr=boolean
  Data Store Write : DataStoreWrite  DataStoreName=VotageReqFreemaster
  FCAN_Receive_ID_0x3FF : mbd_s32k14_ec_toolbox/S32K14x/Communication Blocks/Flex CAN Blocks/FCAN_Receive  can_instance=0  can_mode=Non-blocking  can_timeout_ms=0  can_mb_idx=14  can_extended_id=off  can_is_remote=off  can_id=3FF  can_msg_mask=FFFFFFFF  show_adv_opts=on  can_use_rxfifo=off  can_fd_enable=on
  Relay_Actuation : mbd_s32k14_ec_toolbox/S32K14x/Peripheral Interface Blocks/Digital_Output  gpio_pin=PTD1 : [3] : [1] : [B1]  port=D  pin=1  drive_strength=Low  slew_rate=Fast
  wires:
  Constant/1 -> Data Store Write/1
  Constant1/1 -> Relay_Actuation/1

== stateflow chart StepbyStepMotorControl_Slave_SM/TrapezoidalControl/CommutationTableLookup ==
  (junction 5) -> (junction 15) [order 1] : /*If Direction is Negative */
      | [DIRECTION == -1]
  (default) -> (junction 5)
  (junction 15) -> (junction 14) : {
      |    Phase_A = ccwTable[HallState][0];
      |    Phase_B = ccwTable[HallState][1];
      |    Phase_C = ccwTable[HallState][2];
      | }
  (junction 5) -> (junction 6) [order 2] : {
      |    Phase_A = cwTable[HallState][0];
      |    Phase_B = cwTable[HallState][1];
      |    Phase_C = cwTable[HallState][2];
      | }
  (junction 6) -> (junction 14)
  data: cwTable constant uint8 size=[8 3] =[0 0 0; 2 1 0; 0 2 1; 2 0 1; 1 0 2; 0 1 2; 1 2 0; 0 0 0]; HallState input uint8; Phase_A output uint8; Phase_B output uint8; Phase_C output uint8; ccwTable constant uint8 size=[8 3] =[0 0 0; 1 2 0; 0 1 2; 1 0 2; 2 0 1; 0 2 1; 2 1 0; 0 0 0]; DIRECTION input single

== stateflow chart StepbyStepMotorControl_Slave_SM/Hall_Emulator/DriveCW_or_CCW_HallStateEmulator ==
  state STEP1
    entry:
    hall_A = uint8(1);
    hall_B = uint8(0);
    hall_C = uint8(0);
  state STEP2_CCW
    entry:
    hall_A = uint8(1);
    hall_B = uint8(0);
    hall_C = uint8(1);
  state STEP2_CW
    entry:
    hall_A = uint8(1);
    hall_B = uint8(1);
    hall_C = uint8(0);
  state STEP3_CCW
    entry:
    hall_A = uint8(0);
    hall_B = uint8(0);
    hall_C = uint8(1);
  state STEP3
    entry:
    hall_A = uint8(0);
    hall_B = uint8(1);
    hall_C = uint8(0);
  state STEP4_CCW
    entry:
    hall_A = uint8(0);
    hall_B = uint8(1);
    hall_C = uint8(1);
  state STEP4
    entry:
    hall_A = uint8(0);
    hall_B = uint8(1);
    hall_C = uint8(1);
  state STEP5_CCW
    entry:
    hall_A = uint8(0);
    hall_B = uint8(1);
    hall_C = uint8(0);
  state STEP5
    entry:
    hall_A = uint8(0);
    hall_B = uint8(0);
    hall_C = uint8(1);
  state STEP6_CCW
    entry:
    hall_A = uint8(1);
    hall_B = uint8(1);
    hall_C = uint8(0);
  state STEP6
    entry:
    hall_A = uint8(1);
    hall_B = uint8(0);
    hall_C = uint8(1);
  (default) -> STEP1
  STEP1 -> STEP2_CW [order 1] : [DIRECTION >=0]
  STEP1 -> STEP2_CCW [order 2] : [DIRECTION<0]
  STEP6_CCW -> STEP1
  STEP6 -> STEP1
  STEP2_CW -> STEP3
  STEP2_CCW -> STEP3_CCW
  STEP3_CCW -> STEP4_CCW
  STEP3 -> STEP4
  STEP4_CCW -> STEP5_CCW
  STEP4 -> STEP5
  STEP5_CCW -> STEP6_CCW
  STEP5 -> STEP6
  data: hall_A output uint8; hall_B output uint8; hall_C output uint8; DIRECTION input int16

== stateflow chart StepbyStepMotorControl_Slave_SM/TrapezoidalControl/PhaseSwitchLogic ==
  settings: sampleTime=0.500
  note: Phase States:
      | 0 = NC
      | 1 = -Vdcb
      | 2 = +Vdcb
  (default) -> (junction 13)
  (junction 13) -> (junction 14) [order 1] : /*check for phase state 0 */
      | [Phase_A == 0]
      | /*set output for state 0 */
      | {Phase_A_HS = 0; Phase_A_LS =0;}
  (junction 13) -> (junction 17) [order 2]
  (junction 14) -> (junction 16)
  (junction 17) -> (junction 16) [order 1] : /*check for phase state 1 */
      | [Phase_A == 1]
      | /*set output for state 1 */
      | {Phase_A_HS = 0; Phase_A_LS = PWM_Duty_Cycle;}
  (junction 17) -> (junction 20) [order 2]
  (junction 16) -> (junction 19)
  (junction 20) -> (junction 19) [order 1] : /*check for phase state 2 */
      | [Phase_A == 2]
      | /*set output for state 2 */
      | {Phase_A_HS = 100; Phase_A_LS = 0;}
  (junction 20) -> (junction 62) [order 2]
  (junction 19) -> (junction 23)
  (junction 62) -> (junction 23)
  (junction 23) -> (junction 22) [order 1] : /*check for phase state 0 */
      | [Phase_B == 0]
      | /*set output for state 0 */
      | {Phase_B_HS = 0; Phase_B_LS = 0;}
  (junction 23) -> (junction 26) [order 2]
  (junction 22) -> (junction 25)
  (junction 26) -> (junction 25) [order 1] : /*check for phase state 1 */
      | [Phase_B == 1]
      | /*set output for state 1 */
      | {Phase_B_HS = 0; Phase_B_LS = PWM_Duty_Cycle;}
  (junction 26) -> (junction 29) [order 2]
  (junction 25) -> (junction 28)
  (junction 29) -> (junction 28) [order 1] : /*check for phase state 2 */
      | [Phase_B == 2]
      | /*set output for state 2 */
      | {Phase_B_HS = 100; Phase_B_LS = 0;}
  (junction 29) -> (junction 65) [order 2]
  (junction 28) -> (junction 49)
  (junction 65) -> (junction 49)
  (junction 49) -> (junction 48) [order 1] : /*check for phase state 0 */
      | [Phase_C == 0]
      | /*set output for state 0 */
      | {Phase_C_HS = 0; Phase_C_LS = 0;}
  (junction 49) -> (junction 51) [order 2]
  (junction 48) -> (junction 50)
  (junction 51) -> (junction 50) [order 1] : /*check for phase state 1 */
      | [Phase_C == 1]
      | /*set output for state 1 */
      | {Phase_C_HS = 0; Phase_C_LS = PWM_Duty_Cycle;}
  (junction 51) -> (junction 53) [order 2]
  (junction 50) -> (junction 52)
  (junction 53) -> (junction 52) [order 1] : /*check for phase state 2 */
      | [Phase_C == 2]
      | /*set output for state 2 */
      | {Phase_C_HS = 100; Phase_C_LS = 0;}
  (junction 53) -> (junction 70) [order 2]
  (junction 52) -> (junction 69)
  (junction 70) -> (junction 69)
  data: Phase_A input; Phase_B input; Phase_C input; Phase_A_HS output uint32; Phase_A_LS output uint32; Phase_B_HS output uint32; Phase_B_LS output uint32; Phase_C_HS output uint32; Phase_C_LS output uint32; PWM_Duty_Cycle input
